simulink model "s2"  (Simulink 2.00)
settings: Solver=ode45  StartTime=0.0  StopTime=tstop  MaxStep=0.04  RelTol=1e-6  AbsTol=1e-6
values from neighbouring files (symbols this model uses):
  AEx = 0.0012    [I3ESSR.M]    (also in SET1.M)
  BEx = 1.264    [I3ESSR.M]    (also in SET1.M)
  delio = x(3)    [M1.M]    (also in M3.M = delta4; M3G.M = delta4; M4.M = delta)
  Domega = 0    [I3ESSR.M]    (also in M3.M; M3G.M; M5.M = 1; SET1.M = 2)
  Edpo = x(2)    [M1.M]    (also in M4.M = Vdo - xpq*Iqo + rs*Ido)
  Eqpo = x(1)    [M1.M]    (also in M4.M = Vqo + xpd*Ido + rs*Iqo)
  H = 2.89    [I3ESSR.M]    (also in M1.M = 0.5*J_rotor*wbasem*wbasem/Sbase; M3.M = diag(h); M3G.M = diag(h); M5.M = 0.352825293175)
  KA = 50    [I3ESSR.M]    (also in SET1.M)
  KE = -0.0465    [I3ESSR.M]    (also in SET1.M)
  KF = 0.0832    [I3ESSR.M]    (also in SET1.M)
  rs = 0.00    (= 0)    [I3ESSR.M]    (also in M1.M = rs/Zbase; M3.M; M3G.M = 0.001; M5.M = rs/Zb)
  TA = .06    (= 0.06)    [I3ESSR.M]    (also in SET1.M)
  TE = 0.052    [I3ESSR.M]    (also in SET1.M)
  TF = 1.0    (= 1)    [I3ESSR.M]    (also in SET1.M)
  Tmech = Pemo    [M1.M]    (also in M3.M; M3G.M)
  Tpdo = 4.3    [I3ESSR.M]    (also in SET1.M = 7.9)
  Tpqo = 0.85    [I3ESSR.M]    (also in SET1.M = 0.41)
  VR = KE*Efo    [M4.M]
  VRmax = 1    [I3ESSR.M]    (also in SET1.M)
  VRmin = -1    [I3ESSR.M]    (also in SET1.M)
  Vs = Efo*KF/TF    [M4.M]
  wb = wbase    [M1.M]    (also in M2.M = 376.991118431; M3.M = 376.991118431; M3G.M = 376.991118431; M4.M = we)
  xd = 1.79    [I3ESSR.M]    (also in M1.M = xd/Zbase; M3.M; M3G.M; M5.M = xd/Zb)
  xpd = 0.169    [I3ESSR.M]    (also in M1.M = xpd/Zbase; SET1.M = 0.355)
  xq = 1.71    [I3ESSR.M]    (also in M1.M = xq/Zbase; M3.M; M3G.M; M5.M = xq/Zb)
undefined symbols (not defined in the file or in its folder): Ef, Exc_sw, Sbratio, vref
settings Model: SaveTime=off  SaveOutput=off  ConsistencyChecking=off

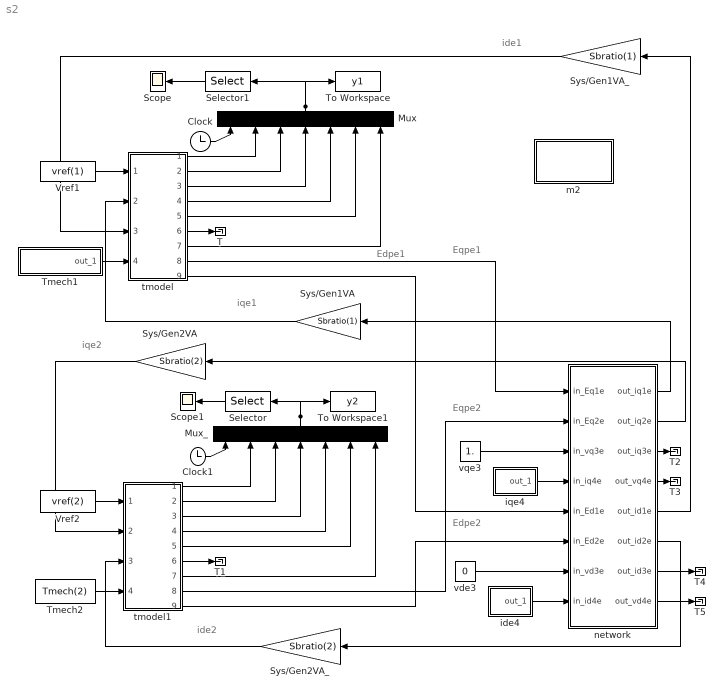
== system s2 ==
  note: Edpe1
  note: Eqpe1
  note: Eqpe2
  note: Edpe2
  note: ide1
  note: iqe1
  note: iqe2
  note: ide2
  Clock : Clock
      settings: DeleteFcn=simclock BlockIsBeingDestroyed  PostSaveFcn=simclock Save
  Clock1 : Clock
      settings: DeleteFcn=simclock BlockIsBeingDestroyed  PostSaveFcn=simclock Save
  m2 : Subsystem
      settings: OpenFcn=m2
      mask Type: Masked block of m2.m
      mask Help: Uses M1.m to initialize and plot
      mask Display: disp('Initialize\nand plot')
  Mux : Mux  Orientation=up  Inputs=7
  Mux_ : Mux  Orientation=up  Inputs=7
  Scope : Scope
      settings: TickLabels=on  TimeRange=20  YMin=-2  YMax=2  SaveToWorkspace=off  SaveName=ScopeData  LimitMaxRows=off
  Scope1 : Scope
      settings: TickLabels=on  TimeRange=20  YMin=-2  YMax=2  SaveToWorkspace=off  SaveName=ScopeData  LimitMaxRows=off
  Selector : Selector  Orientation=left  Elements=[2 3 4 5 6 7]  InputPortWidth=7
  Selector1 : Selector  Orientation=left  Elements=[2 3 4 5 6 7]  InputPortWidth=7
  Sys/Gen1VA : Gain  Orientation=left  Gain=Sbratio(1)
  Sys/Gen1VA_ : Gain  Orientation=left  Gain=Sbratio(1)
  Sys/Gen2VA : Gain  Orientation=left  Gain=Sbratio(2)
  Sys/Gen2VA_ : Gain  Orientation=left  Gain=Sbratio(2)
  T{,1..5} (6 alike) : Terminator
  Tmech1 : Subsystem  mask(Repeating table){@1=time_tmech1, @2=tmech_tmech1}
      mask prompts: @1 "Time values:"; @2 "Output values:"
      mask help:
      | Repeating table.
      | Enter values of time and output for first cycle.
      mask init:
      | period = max(@1); t = @1; y = @2;
      mask Help: Repeats cycle given in table. Time values should be monotonically increasing.
      mask Display: plot([t,t+period,t+2*period],[y,y,y])
  Tmech2 : Constant  Value=Tmech(2)
  To Workspace : ToWorkspace  VariableName=y1  SampleTime=0
      settings: Buffer=40000
  To Workspace1 : ToWorkspace  VariableName=y2  SampleTime=0
      settings: Buffer=240000
  Vref1 : Constant  Value=vref(1)
  Vref2 : Constant  Value=vref(2)
  ide4 : Subsystem  mask(Repeating table){@1=time_id4e, @2=id_id4e}
      mask prompts: @1 "Time values:"; @2 "Output values:"
      mask help:
      | Repeating table.
      | Enter values of time and output for first cycle.
      mask init:
      | period = max(@1); t = @1; y = @2;
      mask Help: Repeats cycle given in table. Time values should be monotonically increasing.
      mask Display: plot([t,t+period,t+2*period],[y,y,y])
  iqe4 : Subsystem  mask(Repeating table){@1=time_iq4e, @2=iq_iq4e}
      mask prompts: @1 "Time values:"; @2 "Output values:"
      mask help:
      | Repeating table.
      | Enter values of time and output for first cycle.
      mask init:
      | period = max(@1); t = @1; y = @2;
      mask Help: Repeats cycle given in table. Time values should be monotonically increasing.
      mask Display: plot([t,t+period,t+2*period],[y,y,y])
  network : Subsystem
  tmodel : Subsystem
  tmodel1 : Subsystem
  vde3 : Constant  Value=0
  vqe3 : Constant  Value=1.
  wires:
  Mux/1 -> Selector1/1, To Workspace/1
  Selector1/1 -> Scope/1
  Mux_/1 -> Selector/1, To Workspace1/1
  Selector/1 -> Scope1/1
  network/4(out_vq4e) -> T3/1
  network/8(out_vd4e) -> T5/1
  network/7(out_id3e) -> T4/1
  network/3(out_iq3e) -> T2/1
  tmodel1/6(out_puslip) -> T1/1
  tmodel/6(out_puslip) -> T/1
  Vref1/1 -> tmodel/1(in_Vref)
  Tmech2/1 -> tmodel1/4(in_Tmech)
  Vref2/1 -> tmodel1/1(in_Vref)
  tmodel/8(out_Eqpe) -> network/1(in_Eq1e)
  tmodel1/8(out_Eqpe) -> network/2(in_Eq2e)
  vqe3/1 -> network/3(in_vq3e)
  iqe4/1(out_1) -> network/4(in_iq4e)
  vde3/1 -> network/7(in_vd3e)
  ide4/1(out_1) -> network/8(in_id4e)
  tmodel/9(out_Edpe) -> network/5(in_Ed1e)
  tmodel1/9(out_Edpe) -> network/6(in_Ed2e)
  Clock/1 -> Mux/1
  tmodel/1(out_|Vt|) -> Mux/2
  tmodel/2(out_|I|) -> Mux/3
  tmodel/3(out_Pgen) -> Mux/4
  tmodel/4(out_Qgen) -> Mux/5
  tmodel/5(out_delta) -> Mux/6
  tmodel/7(out_Tem) -> Mux/7
  Clock1/1 -> Mux_/1
  tmodel1/1(out_|Vt|) -> Mux_/2
  tmodel1/2(out_|I|) -> Mux_/3
  tmodel1/3(out_Pgen) -> Mux_/4
  tmodel1/4(out_Qgen) -> Mux_/5
  tmodel1/5(out_delta) -> Mux_/6
  tmodel1/7(out_Tem) -> Mux_/7
  Tmech1/1(out_1) -> tmodel/4(in_Tmech)
  network/2(out_iq2e) -> Sys/Gen2VA/1
  Sys/Gen2VA/1 -> tmodel1/2(in_iqe)
  Sys/Gen2VA_/1 -> tmodel1/3(in_ide)
  network/6(out_id2e) -> Sys/Gen2VA_/1
  network/1(out_iq1e) -> Sys/Gen1VA/1
  Sys/Gen1VA/1 -> tmodel/2(in_iqe)
  network/5(out_id1e) -> Sys/Gen1VA_/1
  Sys/Gen1VA_/1 -> tmodel/3(in_ide)

== system s2/m2 ==
  note: Masked block uses m2.m
      | to initialize s2.m.

== system s2/Tmech1 ==
  Clock : Clock
      settings: DeleteFcn=simclock BlockIsBeingDestroyed  PostSaveFcn=simclock Save
  Fcn1 : Fcn  Expr=rem(u[1],period)
  Look-Up Table : Lookup  InputValues=t  OutputValues=y
  out_1 : Outport  Port=1  InitialOutput=0
  wires:
  Look-Up Table/1 -> out_1/1
  Clock/1 -> Fcn1/1
  Fcn1/1 -> Look-Up Table/1

== system s2/ide4 ==
  Clock : Clock
      settings: DeleteFcn=simclock BlockIsBeingDestroyed  PostSaveFcn=simclock Save
  Fcn1 : Fcn  Expr=rem(u[1],period)
  Look-Up Table : Lookup  InputValues=t  OutputValues=y
  out_1 : Outport  Port=1  InitialOutput=0
  wires:
  Fcn1/1 -> Look-Up Table/1
  Clock/1 -> Fcn1/1
  Look-Up Table/1 -> out_1/1

== system s2/iqe4 ==
  Clock : Clock
      settings: DeleteFcn=simclock BlockIsBeingDestroyed  PostSaveFcn=simclock Save
  Fcn1 : Fcn  Expr=rem(u[1],period)
  Look-Up Table : Lookup  InputValues=t  OutputValues=y
  out_1 : Outport  Port=1  InitialOutput=0
  wires:
  Fcn1/1 -> Look-Up Table/1
  Clock/1 -> Fcn1/1
  Look-Up Table/1 -> out_1/1

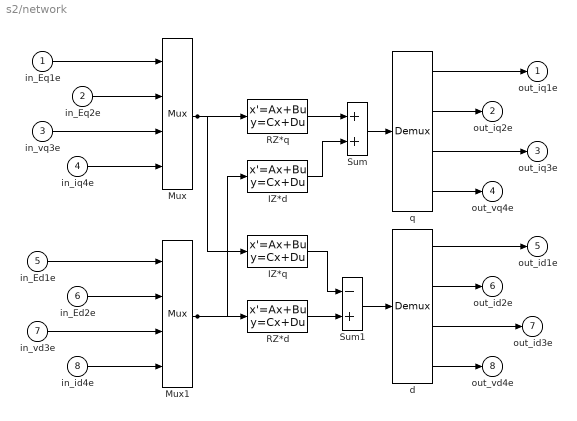
== system s2/network ==
  in_Eq1e : Inport  Port=1  PortWidth=-1  SampleTime=-1
  in_Eq2e : Inport  Port=2  PortWidth=-1  SampleTime=-1
  in_vq3e : Inport  Port=3  PortWidth=-1  SampleTime=-1
  in_iq4e : Inport  Port=4  PortWidth=-1  SampleTime=-1
  in_Ed1e : Inport  Port=5  PortWidth=-1  SampleTime=-1
  in_Ed2e : Inport  Port=6  PortWidth=-1  SampleTime=-1
  in_vd3e : Inport  Port=7  PortWidth=-1  SampleTime=-1
  in_id4e : Inport  Port=8  PortWidth=-1  SampleTime=-1
  IZ*d : StateSpace  A=[]  B=[]  C=[]  D=K  X0=0  mask(Matrix Gain){@1=IZ}
      mask prompts: @1 "Gain matrix:"
      mask help: Matrix Gain.
      mask init:
      | K = @1;
      mask Help: Multiplies input vector by entered matrix to produce output vector (y=Au).
      mask Display: disp('K')
  IZ*q : StateSpace  A=[]  B=[]  C=[]  D=K  X0=0  mask(Matrix Gain){@1=IZ}
      mask prompts: @1 "Gain matrix:"
      mask help: Matrix Gain.
      mask init:
      | K = @1;
      mask Help: Multiplies input vector by entered matrix to produce output vector (y=Au).
      mask Display: disp('K')
  Mux : Mux  Inputs=4
  Mux1 : Mux  Inputs=4
  RZ*d : StateSpace  A=[]  B=[]  C=[]  D=K  X0=0  mask(Matrix Gain){@1=RZ}
      mask prompts: @1 "Gain matrix:"
      mask help: Matrix Gain.
      mask init:
      | K = @1;
      mask Help: Multiplies input vector by entered matrix to produce output vector (y=Au).
      mask Display: disp('K')
  RZ*q : StateSpace  A=[]  B=[]  C=[]  D=K  X0=0  mask(Matrix Gain){@1=RZ}
      mask prompts: @1 "Gain matrix:"
      mask help: Matrix Gain.
      mask init:
      | K = @1;
      mask Help: Multiplies input vector by entered matrix to produce output vector (y=Au).
      mask Display: disp('K')
  Sum : Sum  Inputs=++
  Sum1 : Sum  Inputs=-+
  d : Demux  Outputs=4
  q : Demux  Outputs=4
  out_iq1e : Outport  Port=1  InitialOutput=0
  out_iq2e : Outport  Port=2  InitialOutput=0
  out_iq3e : Outport  Port=3  InitialOutput=0
  out_vq4e : Outport  Port=4  InitialOutput=0
  out_id1e : Outport  Port=5  InitialOutput=0
  out_id2e : Outport  Port=6  InitialOutput=0
  out_id3e : Outport  Port=7  InitialOutput=0
  out_vd4e : Outport  Port=8  InitialOutput=0
  wires:
  Sum1/1 -> d/1
  Sum/1 -> q/1
  RZ*d/1 -> Sum1/2
  IZ*q/1 -> Sum1/1
  IZ*d/1 -> Sum/2
  RZ*q/1 -> Sum/1
  Mux1/1 -> RZ*d/1, IZ*d/1
  Mux/1 -> IZ*q/1, RZ*q/1
  q/1 -> out_iq1e/1
  q/3 -> out_iq3e/1
  q/4 -> out_vq4e/1
  in_Eq2e/1 -> Mux/2
  q/2 -> out_iq2e/1
  d/1 -> out_id1e/1
  d/3 -> out_id3e/1
  d/4 -> out_vd4e/1
  d/2 -> out_id2e/1
  in_Eq1e/1 -> Mux/1
  in_vq3e/1 -> Mux/3
  in_iq4e/1 -> Mux/4
  in_Ed1e/1 -> Mux1/1
  in_Ed2e/1 -> Mux1/2
  in_vd3e/1 -> Mux1/3
  in_id4e/1 -> Mux1/4

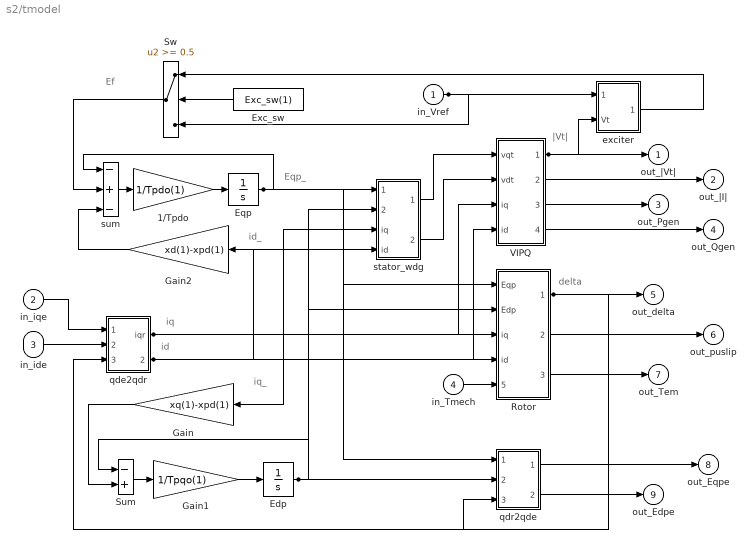
== system s2/tmodel ==
  note: Eqp_
  note: |Vt|
  note: iq_
  note: id_
  note: iq
  note: id
  note: delta
  note: Ef
  in_Vref : Inport  Port=1  PortWidth=-1  SampleTime=-1
  in_iqe : Inport  Port=2  PortWidth=-1  SampleTime=-1
  in_ide : Inport  Port=3  PortWidth=-1  SampleTime=-1
  in_Tmech : Inport  Port=4  PortWidth=-1  SampleTime=-1
  1/Tpdo : Gain  Gain=1/Tpdo(1)
  Edp : Integrator  ExternalReset=none  InitialConditionSource=internal  InitialCondition=Edpo(1)  LimitOutput=off  UpperSaturationLimit=inf  LowerSaturationLimit=-inf  ShowSaturationPort=off  ShowStatePort=off  AbsoluteTolerance=auto
  Eqp : Integrator  ExternalReset=none  InitialConditionSource=internal  InitialCondition=Eqpo(1)  LimitOutput=off  UpperSaturationLimit=inf  LowerSaturationLimit=-inf  ShowSaturationPort=off  ShowStatePort=off  AbsoluteTolerance=auto
  Exc_sw : Constant  Orientation=left  Value=Exc_sw(1)
  Gain : Gain  Orientation=left  Gain=xq(1)-xpd(1)
  Gain1 : Gain  Gain=1/Tpqo(1)
  Gain2 : Gain  Orientation=left  Gain=xd(1)-xpd(1)
  Rotor : Subsystem
  Sum : Sum  Inputs=-+
  Sw : Switch  Orientation=left  Threshold=0.5
  VIPQ : Subsystem
  exciter : Subsystem
  qde2qdr : Subsystem
  qdr2qde : Subsystem
  stator_wdg : Subsystem
  sum : Sum  Inputs=-+-
  out_|Vt| : Outport  Port=1  InitialOutput=0
  out_|I| : Outport  Port=2  InitialOutput=0
  out_Pgen : Outport  Port=3  InitialOutput=0
  out_Qgen : Outport  Port=4  InitialOutput=0
  out_delta : Outport  Port=5  InitialOutput=0
  out_puslip : Outport  Port=6  InitialOutput=0
  out_Tem : Outport  Port=7  InitialOutput=0
  out_Eqpe : Outport  Port=8  InitialOutput=0
  out_Edpe : Outport  Port=9  InitialOutput=0
  wires:
  Eqp/1 -> stator_wdg/1(Eqp), Rotor/1(Eqp), sum/1, qdr2qde/1(Eqp)
  1/Tpdo/1 -> Eqp/1
  sum/1 -> 1/Tpdo/1
  Gain2/1 -> sum/3
  exciter/1(out_Ef) -> Sw/1
  Exc_sw/1 -> Sw/2
  Sw/1 -> sum/2
  VIPQ/2(out_|I|) -> out_|I|/1
  VIPQ/3(out_P) -> out_Pgen/1
  VIPQ/4(out_Q) -> out_Qgen/1
  Rotor/1(out_delta) -> qde2qdr/3("delta "), out_delta/1, qdr2qde/3(delta)
  Rotor/2(out_puslip) -> out_puslip/1
  in_iqe/1 -> qde2qdr/1(iqe)
  Rotor/3(Tem) -> out_Tem/1
  stator_wdg/1(out_vqt) -> VIPQ/1(vqt)
  VIPQ/1(out_|Vt|) -> exciter/2(Vt), out_|Vt|/1
  qdr2qde/1(Eqpe) -> out_Eqpe/1
  qdr2qde/2(Edpe) -> out_Edpe/1
  in_Tmech/1 -> Rotor/5(T_mech)
  Gain/1 -> Sum/2
  Edp/1 -> Sum/1, Rotor/2(Edp), stator_wdg/2(Edp), qdr2qde/2(Edp)
  Sum/1 -> Gain1/1
  Gain1/1 -> Edp/1
  qde2qdr/1(iqr) -> Gain/1, Rotor/3(iq), stator_wdg/3(iq), VIPQ/3(iq)
  qde2qdr/2(vdr) -> Gain2/1, Rotor/4(id), stator_wdg/4(id), VIPQ/4(id)
  in_ide/1 -> qde2qdr/2(ide)
  stator_wdg/2(out_vdt) -> VIPQ/2(vdt)
  in_Vref/1 -> exciter/1(Vref), Sw/3

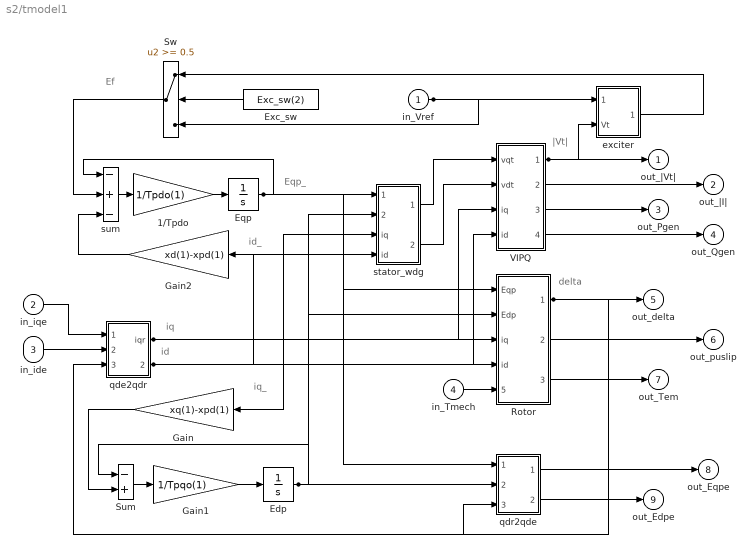
== system s2/tmodel1 ==
  note: Eqp_
  note: |Vt|
  note: Ef
  note: delta
  note: iq_
  note: id_
  note: iq
  note: id
  in_Vref : Inport  Port=1  PortWidth=-1  SampleTime=-1
  in_iqe : Inport  Port=2  PortWidth=-1  SampleTime=-1
  in_ide : Inport  Port=3  PortWidth=-1  SampleTime=-1
  in_Tmech : Inport  Port=4  PortWidth=-1  SampleTime=-1
  1/Tpdo : Gain  Gain=1/Tpdo(1)
  Edp : Integrator  ExternalReset=none  InitialConditionSource=internal  InitialCondition=Edpo(1)  LimitOutput=off  UpperSaturationLimit=inf  LowerSaturationLimit=-inf  ShowSaturationPort=off  ShowStatePort=off  AbsoluteTolerance=auto
  Eqp : Integrator  ExternalReset=none  InitialConditionSource=internal  InitialCondition=Eqpo(1)  LimitOutput=off  UpperSaturationLimit=inf  LowerSaturationLimit=-inf  ShowSaturationPort=off  ShowStatePort=off  AbsoluteTolerance=auto
  Exc_sw : Constant  Orientation=left  Value=Exc_sw(2)
  Gain : Gain  Orientation=left  Gain=xq(1)-xpd(1)
  Gain1 : Gain  Gain=1/Tpqo(1)
  Gain2 : Gain  Orientation=left  Gain=xd(1)-xpd(1)
  Rotor : Subsystem
  Sum : Sum  Inputs=-+
  Sw : Switch  Orientation=left  Threshold=0.5
  VIPQ : Subsystem
  exciter : Subsystem
  qde2qdr : Subsystem
  qdr2qde : Subsystem
  stator_wdg : Subsystem
  sum : Sum  Inputs=-+-
  out_|Vt| : Outport  Port=1  InitialOutput=0
  out_|I| : Outport  Port=2  InitialOutput=0
  out_Pgen : Outport  Port=3  InitialOutput=0
  out_Qgen : Outport  Port=4  InitialOutput=0
  out_delta : Outport  Port=5  InitialOutput=0
  out_puslip : Outport  Port=6  InitialOutput=0
  out_Tem : Outport  Port=7  InitialOutput=0
  out_Eqpe : Outport  Port=8  InitialOutput=0
  out_Edpe : Outport  Port=9  InitialOutput=0
  wires:
  Eqp/1 -> stator_wdg/1(Eqp), Rotor/1(Eqp), sum/1, qdr2qde/1(Eqp)
  1/Tpdo/1 -> Eqp/1
  sum/1 -> 1/Tpdo/1
  Gain2/1 -> sum/3
  exciter/1(out_Ef) -> Sw/1
  Exc_sw/1 -> Sw/2
  Sw/1 -> sum/2
  VIPQ/2(out_|I|) -> out_|I|/1
  VIPQ/3(out_P) -> out_Pgen/1
  VIPQ/4(out_Q) -> out_Qgen/1
  Rotor/1(out_delta) -> qde2qdr/3("delta "), out_delta/1, qdr2qde/3(delta)
  Rotor/2(out_puslip) -> out_puslip/1
  in_iqe/1 -> qde2qdr/1(iqe)
  Rotor/3(Tem) -> out_Tem/1
  stator_wdg/1(out_vqt) -> VIPQ/1(vqt)
  VIPQ/1(out_|Vt|) -> exciter/2(Vt), out_|Vt|/1
  qdr2qde/1(Eqpe) -> out_Eqpe/1
  qdr2qde/2(Edpe) -> out_Edpe/1
  in_Tmech/1 -> Rotor/5(T_mech)
  Gain/1 -> Sum/2
  Edp/1 -> Sum/1, Rotor/2(Edp), stator_wdg/2(Edp), qdr2qde/2(Edp)
  Sum/1 -> Gain1/1
  Gain1/1 -> Edp/1
  qde2qdr/1(iqr) -> Gain/1, Rotor/3(iq), stator_wdg/3(iq), VIPQ/3(iq)
  qde2qdr/2(vdr) -> Gain2/1, Rotor/4(id), stator_wdg/4(id), VIPQ/4(id)
  in_ide/1 -> qde2qdr/2(ide)
  stator_wdg/2(out_vdt) -> VIPQ/2(vdt)
  in_Vref/1 -> exciter/1(Vref), Sw/3

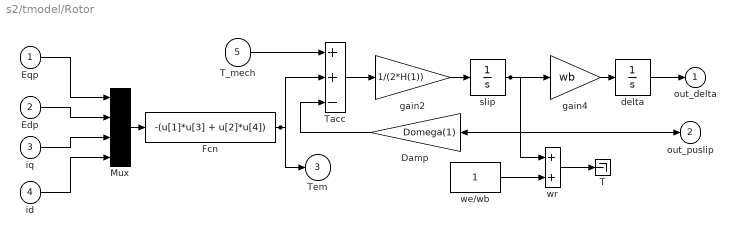
== system s2/tmodel/Rotor ==
  Eqp : Inport  Port=1  PortWidth=-1  SampleTime=-1
  Edp : Inport  Port=2  PortWidth=-1  SampleTime=-1
  iq : Inport  Port=3  PortWidth=-1  SampleTime=-1
  id : Inport  Port=4  PortWidth=-1  SampleTime=-1
  T_mech : Inport  Port=5  PortWidth=-1  SampleTime=-1
  Damp : Gain  Orientation=left  Gain=Domega(1)
  Fcn : Fcn  Expr=-(u[1]*u[3] + u[2]*u[4])
  Mux : Mux  Inputs=4
  T : Terminator
  Tacc : Sum  Inputs=++-
  delta : Integrator  ExternalReset=none  InitialConditionSource=internal  InitialCondition=delio(1)  LimitOutput=off  UpperSaturationLimit=inf  LowerSaturationLimit=-inf  ShowSaturationPort=off  ShowStatePort=off  AbsoluteTolerance=auto
  gain2 : Gain  Gain=1/(2*H(1))
  gain4 : Gain  Gain=wb
  slip : Integrator  ExternalReset=none  InitialConditionSource=internal  InitialCondition=0  LimitOutput=off  UpperSaturationLimit=inf  LowerSaturationLimit=-inf  ShowSaturationPort=off  ShowStatePort=off  AbsoluteTolerance=auto
  we/wb : Constant  Value=1
  wr : Sum  Inputs=++
  out_delta : Outport  Port=1  InitialOutput=0
  out_puslip : Outport  Port=2  InitialOutput=0
  Tem : Outport  Port=3  InitialOutput=0
  wires:
  Damp/1 -> Tacc/3
  T_mech/1 -> Tacc/1
  delta/1 -> out_delta/1
  we/wb/1 -> wr/2
  gain2/1 -> slip/1
  gain4/1 -> delta/1
  slip/1 -> wr/1, out_puslip/1, gain4/1, Damp/1
  Edp/1 -> Mux/2
  Eqp/1 -> Mux/1
  Mux/1 -> Fcn/1
  Fcn/1 -> Tacc/2, Tem/1
  iq/1 -> Mux/3
  id/1 -> Mux/4
  Tacc/1 -> gain2/1
  wr/1 -> T/1

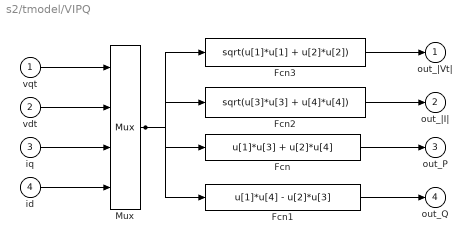
== system s2/tmodel/VIPQ ==
  vqt : Inport  Port=1  PortWidth=-1  SampleTime=-1
  vdt : Inport  Port=2  PortWidth=-1  SampleTime=-1
  iq : Inport  Port=3  PortWidth=-1  SampleTime=-1
  id : Inport  Port=4  PortWidth=-1  SampleTime=-1
  Fcn : Fcn  Expr=u[1]*u[3] + u[2]*u[4]
  Fcn1 : Fcn  Expr=u[1]*u[4] - u[2]*u[3]
  Fcn2 : Fcn  Expr=sqrt(u[3]*u[3] + u[4]*u[4])
  Fcn3 : Fcn  Expr=sqrt(u[1]*u[1] + u[2]*u[2])
  Mux : Mux  Inputs=4
  out_|Vt| : Outport  Port=1  InitialOutput=0
  out_|I| : Outport  Port=2  InitialOutput=0
  out_P : Outport  Port=3  InitialOutput=0
  out_Q : Outport  Port=4  InitialOutput=0
  wires:
  vqt/1 -> Mux/1
  id/1 -> Mux/4
  Fcn/1 -> out_P/1
  Fcn1/1 -> out_Q/1
  Mux/1 -> Fcn/1, Fcn1/1, Fcn3/1, Fcn2/1
  Fcn3/1 -> out_|Vt|/1
  Fcn2/1 -> out_|I|/1
  vdt/1 -> Mux/2
  iq/1 -> Mux/3

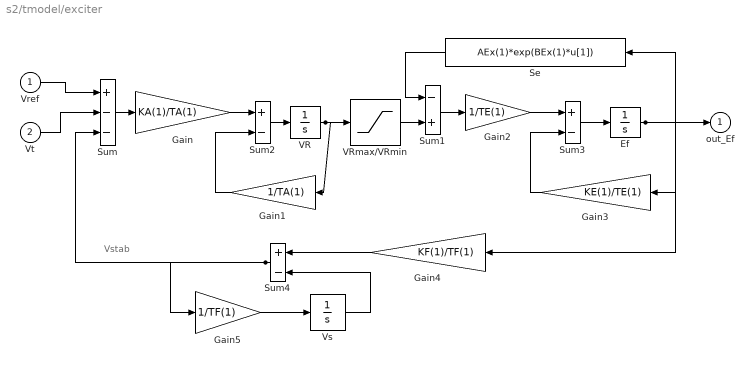
== system s2/tmodel/exciter ==
  note: Vstab
  Vref : Inport  Port=1  PortWidth=-1  SampleTime=-1
  Vt : Inport  Port=2  PortWidth=-1  SampleTime=-1
  Ef : Integrator  ExternalReset=none  InitialConditionSource=internal  InitialCondition=Ef(1)  LimitOutput=off  UpperSaturationLimit=inf  LowerSaturationLimit=-inf  ShowSaturationPort=off  ShowStatePort=off  AbsoluteTolerance=auto
  Gain : Gain  Gain=KA(1)/TA(1)
  Gain1 : Gain  Orientation=left  Gain=1/TA(1)
  Gain2 : Gain  Gain=1/TE(1)
  Gain3 : Gain  Orientation=left  Gain=KE(1)/TE(1)
  Gain4 : Gain  Orientation=left  Gain=KF(1)/TF(1)
  Gain5 : Gain  Gain=1/TF(1)
  Se : Fcn  Orientation=left  Expr=AEx(1)*exp(BEx(1)*u[1])
  Sum : Sum  Inputs=+--
  Sum1 : Sum  Inputs=-+
  Sum2 : Sum  Inputs=+-
  Sum3 : Sum  Inputs=+-
  Sum4 : Sum  Orientation=left  Inputs=+-
  VR : Integrator  ExternalReset=none  InitialConditionSource=internal  InitialCondition=VR(1)  LimitOutput=off  UpperSaturationLimit=inf  LowerSaturationLimit=-inf  ShowSaturationPort=off  ShowStatePort=off  AbsoluteTolerance=auto
  VRmax/VRmin : Saturate  UpperLimit=VRmax(1)  LowerLimit=VRmin(1)
  Vs : Integrator  ExternalReset=none  InitialConditionSource=internal  InitialCondition=Vs(1)  LimitOutput=off  UpperSaturationLimit=inf  LowerSaturationLimit=-inf  ShowSaturationPort=off  ShowStatePort=off  AbsoluteTolerance=auto
  out_Ef : Outport  Port=1  InitialOutput=0
  wires:
  Vt/1 -> Sum/2
  VRmax/VRmin/1 -> Sum1/2
  Vref/1 -> Sum/1
  Se/1 -> Sum1/1
  Sum2/1 -> VR/1
  Sum/1 -> Gain/1
  VR/1 -> VRmax/VRmin/1, Gain1/1
  Sum3/1 -> Ef/1
  Sum1/1 -> Gain2/1
  Gain2/1 -> Sum3/1
  Gain3/1 -> Sum3/2
  Ef/1 -> Gain3/1, Se/1, out_Ef/1, Gain4/1
  Gain/1 -> Sum2/1
  Gain1/1 -> Sum2/2
  Gain4/1 -> Sum4/1
  Gain5/1 -> Vs/1
  Vs/1 -> Sum4/2
  Sum4/1 -> Sum/3, Gain5/1

== system s2/tmodel/qde2qdr ==
  iqe : Inport  Port=1  PortWidth=-1  SampleTime=-1
  ide : Inport  Port=2  PortWidth=-1  SampleTime=-1
  "delta " : Inport  Port=3  PortWidth=-1  SampleTime=-1
  Mux : Mux  Inputs=3
  fcn : Fcn  Expr=u[1]*cos(u[3]) - u[2]*sin(u[3])
  fcn1 : Fcn  Expr=u[1]*sin(u[3]) + u[2]*cos(u[3])
  iqr : Outport  Port=1  InitialOutput=0
  vdr : Outport  Port=2  InitialOutput=0
  wires:
  fcn1/1 -> vdr/1
  iqe/1 -> Mux/1
  fcn/1 -> iqr/1
  Mux/1 -> fcn/1, fcn1/1
  "delta "/1 -> Mux/3
  ide/1 -> Mux/2

== system s2/tmodel/qdr2qde ==
  Eqp : Inport  Port=1  PortWidth=-1  SampleTime=-1
  Edp : Inport  Port=2  PortWidth=-1  SampleTime=-1
  delta : Inport  Port=3  PortWidth=-1  SampleTime=-1
  Mux : Mux  Inputs=3
  fcn : Fcn  Expr=u[1]*cos(u[3]) + u[2]*sin(u[3])
  fcn1 : Fcn  Expr=-u[1]*sin(u[3]) + u[2]*cos(u[3])
  Eqpe : Outport  Port=1  InitialOutput=0
  Edpe : Outport  Port=2  InitialOutput=0
  wires:
  fcn1/1 -> Edpe/1
  Eqp/1 -> Mux/1
  fcn/1 -> Eqpe/1
  Mux/1 -> fcn/1, fcn1/1
  Edp/1 -> Mux/2
  delta/1 -> Mux/3

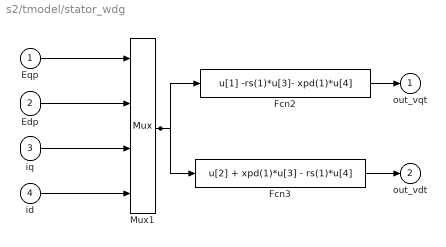
== system s2/tmodel/stator_wdg ==
  Eqp : Inport  Port=1  PortWidth=-1  SampleTime=-1
  Edp : Inport  Port=2  PortWidth=-1  SampleTime=-1
  iq : Inport  Port=3  PortWidth=-1  SampleTime=-1
  id : Inport  Port=4  PortWidth=-1  SampleTime=-1
  Fcn2 : Fcn  Expr=u[1] -rs(1)*u[3]- xpd(1)*u[4]
  Fcn3 : Fcn  Expr=u[2] + xpd(1)*u[3] - rs(1)*u[4]
  Mux1 : Mux  Inputs=4
  out_vqt : Outport  Port=1  InitialOutput=0
  out_vdt : Outport  Port=2  InitialOutput=0
  wires:
  Eqp/1 -> Mux1/1
  Mux1/1 -> Fcn2/1, Fcn3/1
  Fcn2/1 -> out_vqt/1
  Fcn3/1 -> out_vdt/1
  iq/1 -> Mux1/3
  id/1 -> Mux1/4
  Edp/1 -> Mux1/2

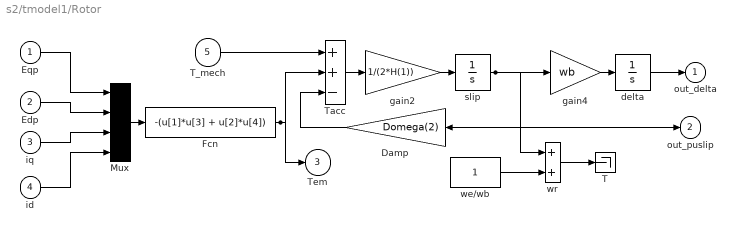
== system s2/tmodel1/Rotor ==
  Eqp : Inport  Port=1  PortWidth=-1  SampleTime=-1
  Edp : Inport  Port=2  PortWidth=-1  SampleTime=-1
  iq : Inport  Port=3  PortWidth=-1  SampleTime=-1
  id : Inport  Port=4  PortWidth=-1  SampleTime=-1
  T_mech : Inport  Port=5  PortWidth=-1  SampleTime=-1
  Damp : Gain  Orientation=left  Gain=Domega(2)
  Fcn : Fcn  Expr=-(u[1]*u[3] + u[2]*u[4])
  Mux : Mux  Inputs=4
  T : Terminator
  Tacc : Sum  Inputs=++-
  delta : Integrator  ExternalReset=none  InitialConditionSource=internal  InitialCondition=delio(1)  LimitOutput=off  UpperSaturationLimit=inf  LowerSaturationLimit=-inf  ShowSaturationPort=off  ShowStatePort=off  AbsoluteTolerance=auto
  gain2 : Gain  Gain=1/(2*H(1))
  gain4 : Gain  Gain=wb
  slip : Integrator  ExternalReset=none  InitialConditionSource=internal  InitialCondition=0  LimitOutput=off  UpperSaturationLimit=inf  LowerSaturationLimit=-inf  ShowSaturationPort=off  ShowStatePort=off  AbsoluteTolerance=auto
  we/wb : Constant  Value=1
  wr : Sum  Inputs=++
  out_delta : Outport  Port=1  InitialOutput=0
  out_puslip : Outport  Port=2  InitialOutput=0
  Tem : Outport  Port=3  InitialOutput=0
  wires:
  Damp/1 -> Tacc/3
  T_mech/1 -> Tacc/1
  delta/1 -> out_delta/1
  we/wb/1 -> wr/2
  gain2/1 -> slip/1
  gain4/1 -> delta/1
  slip/1 -> wr/1, out_puslip/1, gain4/1, Damp/1
  Edp/1 -> Mux/2
  Eqp/1 -> Mux/1
  Mux/1 -> Fcn/1
  Fcn/1 -> Tacc/2, Tem/1
  iq/1 -> Mux/3
  id/1 -> Mux/4
  Tacc/1 -> gain2/1
  wr/1 -> T/1

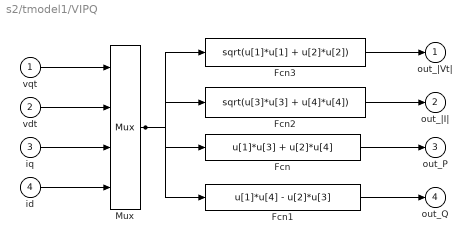
== system s2/tmodel1/VIPQ ==
  vqt : Inport  Port=1  PortWidth=-1  SampleTime=-1
  vdt : Inport  Port=2  PortWidth=-1  SampleTime=-1
  iq : Inport  Port=3  PortWidth=-1  SampleTime=-1
  id : Inport  Port=4  PortWidth=-1  SampleTime=-1
  Fcn : Fcn  Expr=u[1]*u[3] + u[2]*u[4]
  Fcn1 : Fcn  Expr=u[1]*u[4] - u[2]*u[3]
  Fcn2 : Fcn  Expr=sqrt(u[3]*u[3] + u[4]*u[4])
  Fcn3 : Fcn  Expr=sqrt(u[1]*u[1] + u[2]*u[2])
  Mux : Mux  Inputs=4
  out_|Vt| : Outport  Port=1  InitialOutput=0
  out_|I| : Outport  Port=2  InitialOutput=0
  out_P : Outport  Port=3  InitialOutput=0
  out_Q : Outport  Port=4  InitialOutput=0
  wires:
  vqt/1 -> Mux/1
  id/1 -> Mux/4
  Fcn/1 -> out_P/1
  Fcn1/1 -> out_Q/1
  Mux/1 -> Fcn/1, Fcn1/1, Fcn3/1, Fcn2/1
  Fcn3/1 -> out_|Vt|/1
  Fcn2/1 -> out_|I|/1
  vdt/1 -> Mux/2
  iq/1 -> Mux/3

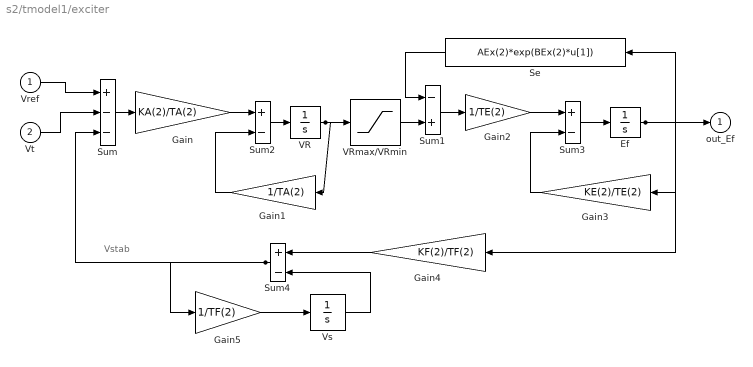
== system s2/tmodel1/exciter ==
  note: Vstab
  Vref : Inport  Port=1  PortWidth=-1  SampleTime=-1
  Vt : Inport  Port=2  PortWidth=-1  SampleTime=-1
  Ef : Integrator  ExternalReset=none  InitialConditionSource=internal  InitialCondition=Ef(2)  LimitOutput=off  UpperSaturationLimit=inf  LowerSaturationLimit=-inf  ShowSaturationPort=off  ShowStatePort=off  AbsoluteTolerance=auto
  Gain : Gain  Gain=KA(2)/TA(2)
  Gain1 : Gain  Orientation=left  Gain=1/TA(2)
  Gain2 : Gain  Gain=1/TE(2)
  Gain3 : Gain  Orientation=left  Gain=KE(2)/TE(2)
  Gain4 : Gain  Orientation=left  Gain=KF(2)/TF(2)
  Gain5 : Gain  Gain=1/TF(2)
  Se : Fcn  Orientation=left  Expr=AEx(2)*exp(BEx(2)*u[1])
  Sum : Sum  Inputs=+--
  Sum1 : Sum  Inputs=-+
  Sum2 : Sum  Inputs=+-
  Sum3 : Sum  Inputs=+-
  Sum4 : Sum  Orientation=left  Inputs=+-
  VR : Integrator  ExternalReset=none  InitialConditionSource=internal  InitialCondition=VR(2)  LimitOutput=off  UpperSaturationLimit=inf  LowerSaturationLimit=-inf  ShowSaturationPort=off  ShowStatePort=off  AbsoluteTolerance=auto
  VRmax/VRmin : Saturate  UpperLimit=VRmax(2)  LowerLimit=VRmin(2)
  Vs : Integrator  ExternalReset=none  InitialConditionSource=internal  InitialCondition=Vs(2)  LimitOutput=off  UpperSaturationLimit=inf  LowerSaturationLimit=-inf  ShowSaturationPort=off  ShowStatePort=off  AbsoluteTolerance=auto
  out_Ef : Outport  Port=1  InitialOutput=0
  wires:
  Vt/1 -> Sum/2
  VRmax/VRmin/1 -> Sum1/2
  Vref/1 -> Sum/1
  Se/1 -> Sum1/1
  Sum2/1 -> VR/1
  Sum/1 -> Gain/1
  VR/1 -> VRmax/VRmin/1, Gain1/1
  Sum3/1 -> Ef/1
  Sum1/1 -> Gain2/1
  Gain2/1 -> Sum3/1
  Gain3/1 -> Sum3/2
  Ef/1 -> Gain3/1, Se/1, out_Ef/1, Gain4/1
  Gain/1 -> Sum2/1
  Gain1/1 -> Sum2/2
  Gain4/1 -> Sum4/1
  Gain5/1 -> Vs/1
  Vs/1 -> Sum4/2
  Sum4/1 -> Sum/3, Gain5/1

== system s2/tmodel1/qde2qdr ==
  iqe : Inport  Port=1  PortWidth=-1  SampleTime=-1
  ide : Inport  Port=2  PortWidth=-1  SampleTime=-1
  "delta " : Inport  Port=3  PortWidth=-1  SampleTime=-1
  Mux : Mux  Inputs=3
  fcn : Fcn  Expr=u[1]*cos(u[3]) - u[2]*sin(u[3])
  fcn1 : Fcn  Expr=u[1]*sin(u[3]) + u[2]*cos(u[3])
  iqr : Outport  Port=1  InitialOutput=0
  vdr : Outport  Port=2  InitialOutput=0
  wires:
  fcn1/1 -> vdr/1
  iqe/1 -> Mux/1
  fcn/1 -> iqr/1
  Mux/1 -> fcn/1, fcn1/1
  "delta "/1 -> Mux/3
  ide/1 -> Mux/2

== system s2/tmodel1/qdr2qde ==
  Eqp : Inport  Port=1  PortWidth=-1  SampleTime=-1
  Edp : Inport  Port=2  PortWidth=-1  SampleTime=-1
  delta : Inport  Port=3  PortWidth=-1  SampleTime=-1
  Mux : Mux  Inputs=3
  fcn : Fcn  Expr=u[1]*cos(u[3]) + u[2]*sin(u[3])
  fcn1 : Fcn  Expr=-u[1]*sin(u[3]) + u[2]*cos(u[3])
  Eqpe : Outport  Port=1  InitialOutput=0
  Edpe : Outport  Port=2  InitialOutput=0
  wires:
  fcn1/1 -> Edpe/1
  Eqp/1 -> Mux/1
  fcn/1 -> Eqpe/1
  Mux/1 -> fcn/1, fcn1/1
  Edp/1 -> Mux/2
  delta/1 -> Mux/3

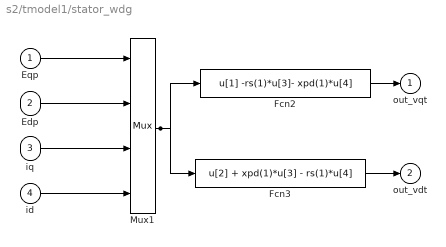
== system s2/tmodel1/stator_wdg ==
  Eqp : Inport  Port=1  PortWidth=-1  SampleTime=-1
  Edp : Inport  Port=2  PortWidth=-1  SampleTime=-1
  iq : Inport  Port=3  PortWidth=-1  SampleTime=-1
  id : Inport  Port=4  PortWidth=-1  SampleTime=-1
  Fcn2 : Fcn  Expr=u[1] -rs(1)*u[3]- xpd(1)*u[4]
  Fcn3 : Fcn  Expr=u[2] + xpd(1)*u[3] - rs(1)*u[4]
  Mux1 : Mux  Inputs=4
  out_vqt : Outport  Port=1  InitialOutput=0
  out_vdt : Outport  Port=2  InitialOutput=0
  wires:
  Eqp/1 -> Mux1/1
  Mux1/1 -> Fcn2/1, Fcn3/1
  Fcn2/1 -> out_vqt/1
  Fcn3/1 -> out_vdt/1
  iq/1 -> Mux1/3
  id/1 -> Mux1/4
  Edp/1 -> Mux1/2
